simulink model "Mission_Server_QDrone_minimal_data"  (R2019a)
settings: Solver=ode2  StartTime=0.0  StopTime=inf  FixedStep=0.001  RelTol=1e-3  EnableMultiTasking=on
undefined symbols (not defined in the file or in its folder): Host, qc_get_step_size
libraries: quarc_library x34, simulink x5
(part 2 of 2)

== matlab function Mission_Server_QDrone_minimal_data/MISSION SERVER QDRONE POSITION CONTROL/min snap Trajectories1/MATLAB Function ==
  data: enable input; x output; time input; y output; z output; yaw output; xdot output; ydot output; zdot output; done output
function [x, y, z, yaw, xdot, ydot, zdot, done]= fcn(enable, time)

persistent start_time
persistent poly_x
persistent poly_y
persistent poly_z
persistent n_order
persistent ts
persistent trajectory_segment
persistent state 
%states:
%   1: First trajectory
%   2: Second trajectory
%   3: Third trajectory


if isempty(start_time) || isempty(trajectory_segment) || ~enable || isempty(state)
    start_time = time;
    trajectory_segment = 1;
    state = 1;
end

if isempty(poly_x) || isempty(poly_y) || isempty(poly_z) || isempty(ts)
    g = coder.load('8shape-15_time_minsnap.mat');
    poly_t = g.y;
    n_order = g.poly_order;
    ts = g.T;
end

T = 5.5;
x = 0; y = 0; z = 1; yaw=0; done=false;
xdot = 0; ydot = 0; zdot = 0; 
if enable
    t = time - start_time;
    if t > T
        x = 0; y = 0; z = 1; yaw = 0; done = true;
        xdot = 0; ydot = 0; zdot = 0; 
        return;
    end
    t_now = 0;
    for i=0:n_order
        t_now = t_now + poly_t(i+1) * t^i;
    end
    t_now = 2*pi*t_now/T - pi/2;
    x = 1*cos(t_now)*sin(t_now);
    y = 1*cos(t_now);
    
end

% 
% 
% if isempty(poly_x) || isempty(poly_y) || isempty(poly_z) || isempty(ts)
%     g = coder.load('90_deg_roll24.mat');
%     poly_x = g.polys_x;
%     poly_y = g.polys_y;
%     poly_z = g.polys_z;
%     n_order = g.n_order(1);
%     ts = g.ts;
% end
% 
% x = -3; y = 0; z = 0.85; yaw=0; done=false;
% xdot = 0; ydot = 0; zdot = 0; 
% if enable
%     t = time - start_time;
%     if t > ts(end)
%         t=ts(end)
%     elseif t > ts(trajectory_segment + 1)
%         trajectory_segment = trajectory_segment + 1;
%     end
% 
% %     poly_x_i = poly_x(:, trajectory_segment);
% %     poly_y_i = poly_y(:, trajectory_segment);
% %     poly_z_i = poly_z(:, trajectory_segment);
%     poly_x_i = poly_x{trajectory_segment};
%     poly_y_i = poly_y{trajectory_segment};
%     poly_z_i = poly_z{trajectory_segment};
% 
%     x = 0; y = 0; z = 0.25;
%     for i=0:n_order
%         x = x + poly_x_i(i+1) * t^i;
%         y = y + poly_y_i(i+1) * t^i;
%         z = z + poly_z_i(i+1) * t^i;
%         if i>0
%             xdot = xdot + i * poly_x_i(i+1) * t^(i-1);
%             ydot = ydot + i * poly_y_i(i+1) * t^(i-1);
%             zdot = zdot + i * poly_z_i(i+1) * t^(i-1);
%         end
%     end
% end


% if isempty(poly_x) || isempty(poly_y) || isempty(poly_z) || isempty(n_order) || isempty(ts)
%     g = coder.load('90_deg_roll24.mat');
%     poly_x = g.polys_x;
%     poly_y = g.polys_y;
%     poly_z = g.polys_z;
%     n_order = g.n_order(1);
%     ts = g.ts;
% end


% x = -3; y = 0; z = 0.75; yaw=0; done=false;
% xdot = 0; ydot = 0; zdot = 0; 
% if enable
%     t = time - start_time; 
%     tt = t;
%     if t > ts(end)
%         tt = ts(end);
%     elseif t > ts(trajectory_segment + 1)
%         trajectory_segment = trajectory_segment + 1;
%     end
% 
% %     poly_x_i = poly_x(:, trajectory_segment);
% %     poly_y_i = poly_y(:, trajectory_segment);
% %     poly_z_i = poly_z(:, trajectory_segment);
%     poly_x_i = poly_x{trajectory_segment};
%     poly_y_i = poly_y{trajectory_segment};
%     poly_z_i = poly_z{trajectory_segment};
% 
%     offset = [0, 0, 0];
%     if state == 1
%         offset = [0, 0, 0.15];
%     elseif state == 2
%         offset = [0, 0, 0.15];
%     elseif state == 3
%         offset = [-0.25, 0.2, 0.25];
%     end
%     x = offset(1); y = offset(2); z = offset(3);
%     for i=0:n_order
%         x = x + poly_x_i(i+1) * tt^i;
%         y = y + poly_y_i(i+1) * tt^i;
%         z = z + poly_z_i(i+1) * tt^i;
%         if i>0
%             xdot = xdot + i * poly_x_i(i+1) * tt^(i-1);
%             ydot = ydot + i * poly_y_i(i+1) * tt^(i-1);
%             zdot = zdot + i * poly_z_i(i+1) * tt^(i-1);
%         end
%     end
%     
%     if t > ts(end)+0.5
%         switch state
%             case 1
%                 state = 2;
%                 start_time = time;
%                 g = coder.load('reset_traj_24_16.mat');
%                 poly_x = g.polys_x;
%                 poly_y = g.polys_y;
%                 poly_z = g.polys_z;
%                 n_order = g.n_order(1);
%                 ts = g.ts;
%                 trajectory_segment = 1;
%             case 2
%                 if t > ts(end)+6
%                     state = 3;
%                     start_time = time;
%                     g = coder.load('90_deg_roll16.mat');                
%                     poly_x = g.polys_x;
%                     poly_y = g.polys_y;
%                     poly_z = g.polys_z;
%                     n_order = g.n_order(1);
%                     ts = g.ts;     
%                     trajectory_segment = 1;       
%                 end
%                 
%         end
%     end
%         
% end

== matlab function Mission_Server_QDrone_minimal_data/MISSION SERVER QDRONE POSITION CONTROL/Extract Vehicle Data/Extract Object Data ==
  data: data input; position output; orientation output; index input; tracking output
function [position, orientation, tracking] = fcn(data, index)

n = length(data)/7;

if (index<=0)||(index>n)
    position = zeros(1,3); orientation = zeros(1,3); tracking = 0;
else
    position = [data(index*3-2), data(index*3-1), data(index*3)];
    orientation = [data((index+n)*3 - 2), data((index+n)*3 - 1), data((index+n)*3)];
    tracking = data(index + (n*6));
end

== matlab function Mission_Server_QDrone_minimal_data/Communication/Detect Communication loss/MATLAB Function ==
  data: time input; stream_connection_loss output; state input; error input
function stream_connection_loss  = fcn(time, state, error)

stream_connection_loss = 0;
if time > 1
    if ~((state == 2)&&(error >= 0))
        % stream connection is not established correctly
        stream_connection_loss = 1;
    end
end

== matlab function Mission_Server_QDrone_minimal_data/MISSION SERVER QDRONE POSITION CONTROL/Data Server (Localization) /Convention Correction (Motive Frame to Research Studio Frame)/MATLAB Function ==
  data: quat_MF input; rpy output; rotmat_RSP_MF input; rot_vec output
function [rpy, rot_vec] = MF_quat_to_RSF_rpy(quat_MF, rotmat_RSP_MF)

MF_drone = quat2rotm([quat_MF(4), quat_MF(1), quat_MF(2), quat_MF(3)]);

corrected_drone_drone = [0 0 -1; -1 0 0 ; 0 1 0];

RSF_drone = rotmat_RSP_MF * MF_drone * corrected_drone_drone';

ypr = rotm2eul(RSF_drone, 'ZYX');

rpy = flip(ypr);

g = trace((trace(RSF_drone) - 1) / 2);
g = min(1, max(g, -1));
theta_error = acos(g);

e_roll = theta_error * ( RSF_drone(3,2) - RSF_drone(2,3) ) / (2 * sin(theta_error));
e_pitch = theta_error * ( RSF_drone(1,3) - RSF_drone(3,1) ) / (2 * sin(theta_error));
e_yaw = theta_error * ( RSF_drone(2,1) - RSF_drone(1,2) ) / (2 * sin(theta_error));

rot_vec = [e_roll, e_pitch, e_yaw];

== matlab function Mission_Server_QDrone_minimal_data/MISSION SERVER QDRONE POSITION CONTROL/Data Server (Localization) with window/Convention Correction (Motive Frame to Research Studio Frame)/MATLAB Function ==
  data: quat_MF input; rpy output; rotmat_RSP_MF input; rot_vec output
function [rpy, rot_vec] = MF_quat_to_RSF_rpy(quat_MF, rotmat_RSP_MF)

MF_drone = quat2rotm([quat_MF(4), quat_MF(1), quat_MF(2), quat_MF(3)]);

corrected_drone_drone = [0 0 -1; -1 0 0 ; 0 1 0];

RSF_drone = rotmat_RSP_MF * MF_drone * corrected_drone_drone';

ypr = rotm2eul(RSF_drone, 'ZYX');

rpy = flip(ypr);

g = trace((trace(RSF_drone) - 1) / 2);
g = min(1, max(g, -1));
theta_error = acos(g);

e_roll = theta_error * ( RSF_drone(3,2) - RSF_drone(2,3) ) / (2 * sin(theta_error));
e_pitch = theta_error * ( RSF_drone(1,3) - RSF_drone(3,1) ) / (2 * sin(theta_error));
e_yaw = theta_error * ( RSF_drone(2,1) - RSF_drone(1,2) ) / (2 * sin(theta_error));

rot_vec = [e_roll, e_pitch, e_yaw];

== matlab function Mission_Server_QDrone_minimal_data/MISSION SERVER QDRONE POSITION CONTROL/Data Server (Localization) with window/Convention Correction/MATLAB Function ==
  data: quat_MF input; rpy output; rotmat_RSP_MF input; rot_vec output
function [rpy, rot_vec] = MF_quat_to_RSF_rpy(quat_MF, rotmat_RSP_MF)

MF_drone = quat2rotm([quat_MF(4), quat_MF(1), quat_MF(2), quat_MF(3)]);

corrected_drone_drone = [0 0 -1; -1 0 0 ; 0 1 0];

RSF_drone = rotmat_RSP_MF * MF_drone * corrected_drone_drone';

ypr = rotm2eul(RSF_drone, 'ZYX');

rpy = flip(ypr);

g = trace((trace(RSF_drone) - 1) / 2);
g = min(1, max(g, -1));
theta_error = acos(g);

e_roll = theta_error * ( RSF_drone(3,2) - RSF_drone(2,3) ) / (2 * sin(theta_error));
e_pitch = theta_error * ( RSF_drone(1,3) - RSF_drone(3,1) ) / (2 * sin(theta_error));
e_yaw = theta_error * ( RSF_drone(2,1) - RSF_drone(1,2) ) / (2 * sin(theta_error));

rot_vec = [e_roll, e_pitch, e_yaw];

== matlab function Mission_Server_QDrone_minimal_data/Communication1/Detect Communication loss/MATLAB Function ==
  data: time input; stream_connection_loss output; state input; error input
function stream_connection_loss  = fcn(time, state, error)

stream_connection_loss = 0;
if time > 1
    if ~((state == 2)&&(error >= 0))
        % stream connection is not established correctly
        stream_connection_loss = 1;
    end
end
